simulink model "linear_simulation"  (R2023a)
settings: Solver=VariableStepAuto  StartTime=0.0  StopTime=10  RelTol=1e-3
undefined symbols (not defined in the file): A_num, b_num, c, init_cond, Ts
libraries: simulink x1
settings Model: Creator=ninj2  LastModifiedBy=morit
settings OptimizationCC: ReuseModelBlockBuffer=off

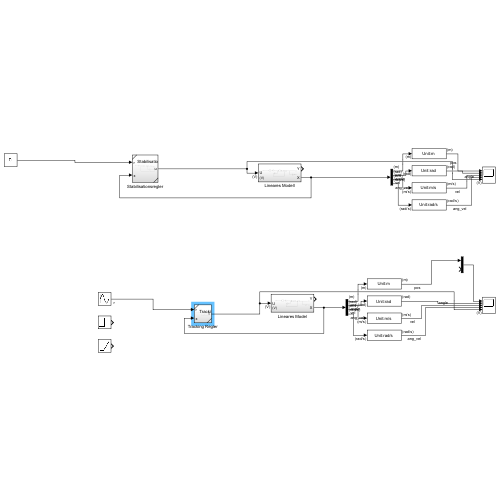
[thumbnail: Simulink's stored preview of the top-level diagram]
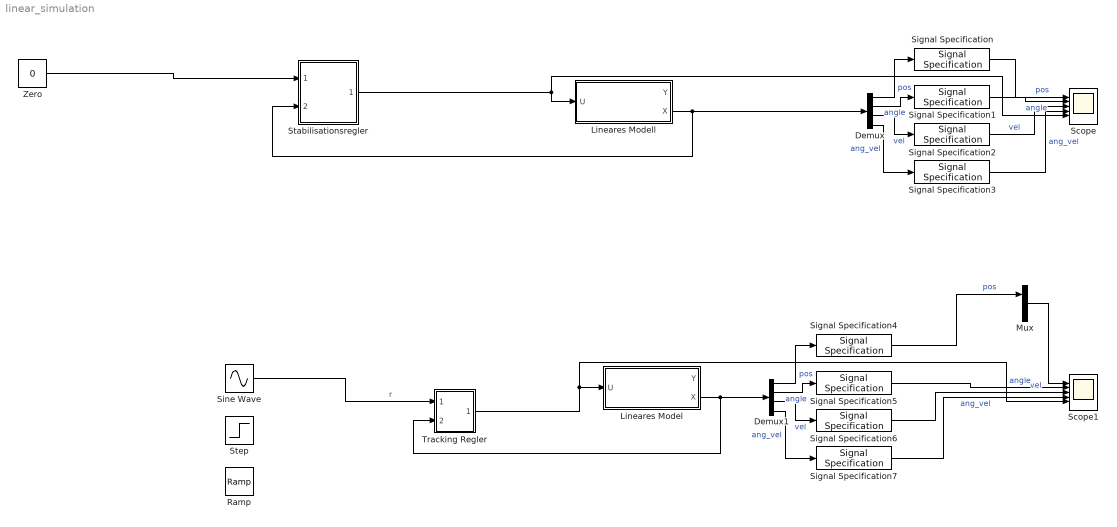
== system linear_simulation ==
  Demux : Demux
  Demux1 : Demux
  Lineares Model : Subsystem
  Lineares Modell : Subsystem
  Mux : Mux  Inputs=2
  Ramp : simulink/Sources/Ramp  slope=0.01  start=0  InitialOutput=0
  Scope : Scope  NumInputPorts=5
  Scope1 : Scope  NumInputPorts=5
  Signal Specification : SignalSpecification  Unit=m
  Signal Specification1 : SignalSpecification  Unit=rad
  Signal Specification2 : SignalSpecification  Unit=m/s
  Signal Specification3 : SignalSpecification  Unit=rad/s
  Signal Specification4 : SignalSpecification  Unit=m
  Signal Specification5 : SignalSpecification  Unit=rad
  Signal Specification6 : SignalSpecification  Unit=m/s
  Signal Specification7 : SignalSpecification  Unit=rad/s
  Sine Wave : Sin  Amplitude=0.05  Frequency=0.3  SampleTime=0
  Stabilisationsregler : Subsystem  ReferencedSubsystem=Stabilisationsregler
  Step : Step  After=0.05  SampleTime=0
  Tracking Regler : Subsystem  ReferencedSubsystem=Tracking_Regler
  Zero : Constant  Value=0  OutDataTypeStr=Inherit: Inherit via back propagation
  wires:
  Lineares Modell/2(X) -> Stabilisationsregler/2, Demux/1
  Demux/1 -> Signal Specification/1  "pos"
  Demux/2 -> Signal Specification1/1  "angle"
  Demux/3 -> Signal Specification2/1  "vel"
  Demux/4 -> Signal Specification3/1  "ang_vel"
  Signal Specification/1 -> Scope/1  "pos"
  Signal Specification1/1 -> Scope/2  "angle"
  Signal Specification2/1 -> Scope/3  "vel"
  Signal Specification3/1 -> Scope/4  "ang_vel"
  Demux1/1 -> Signal Specification4/1  "pos"
  Signal Specification7/1 -> Scope1/4  "ang_vel"
  Signal Specification6/1 -> Scope1/3  "vel"
  Demux1/3 -> Signal Specification6/1  "vel"
  Signal Specification4/1 -> Mux/1  "pos"
  Demux1/4 -> Signal Specification7/1  "ang_vel"
  Signal Specification5/1 -> Scope1/2  "angle"
  Lineares Model/2(X) -> Tracking Regler/2, Demux1/1
  Demux1/2 -> Signal Specification5/1  "angle"
  Mux/1 -> Scope1/1
  Stabilisationsregler/1 -> Lineares Modell/1(U), Scope/5
  Zero/1 -> Stabilisationsregler/1
  Tracking Regler/1 -> Scope1/5, Lineares Model/1(U)
  Sine Wave/1 -> Tracking Regler/1  "r"

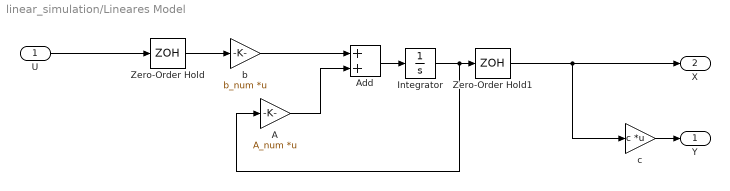
== system linear_simulation/Lineares Model ==
  U : Inport  Unit=V
  A : Gain  Gain=A_num  Multiplication=Matrix(K*u)
  Add : Sum
  Integrator : Integrator  InitialCondition=init_cond
  Zero-Order Hold : ZeroOrderHold  SampleTime=Ts
  Zero-Order Hold1 : ZeroOrderHold  SampleTime=Ts
  b : Gain  Gain=b_num  Multiplication=Matrix(K*u)
  c : Gain  Gain=c  Multiplication=Matrix(K*u)
  Y : Outport
  X : Outport  Port=2
  wires:
  A/1 -> Add/2
  Add/1 -> Integrator/1
  Integrator/1 -> A/1, Zero-Order Hold1/1
  c/1 -> Y/1
  Zero-Order Hold/1 -> b/1
  b/1 -> Add/1
  Zero-Order Hold1/1 -> c/1, X/1
  U/1 -> Zero-Order Hold/1

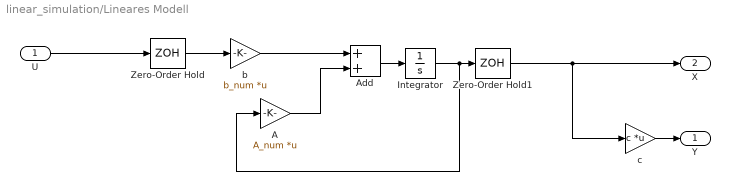
== system linear_simulation/Lineares Modell ==
  U : Inport  Unit=V
  A : Gain  Gain=A_num  Multiplication=Matrix(K*u)
  Add : Sum
  Integrator : Integrator  InitialCondition=init_cond
  Zero-Order Hold : ZeroOrderHold  SampleTime=Ts
  Zero-Order Hold1 : ZeroOrderHold  SampleTime=Ts
  b : Gain  Gain=b_num  Multiplication=Matrix(K*u)
  c : Gain  Gain=c  Multiplication=Matrix(K*u)
  Y : Outport
  X : Outport  Port=2
  wires:
  A/1 -> Add/2
  Add/1 -> Integrator/1
  Integrator/1 -> A/1, Zero-Order Hold1/1
  c/1 -> Y/1
  Zero-Order Hold/1 -> b/1
  b/1 -> Add/1
  Zero-Order Hold1/1 -> c/1, X/1
  U/1 -> Zero-Order Hold/1
